simulink model "BungeeJumpingDragSoln"  (R2024a)
settings: Solver=VariableStepAuto  StartTime=0.0  StopTime=50  MaxStep=0.1  RelTol=1e-3
PreLoadFcn:
  | load Data\BungeeParamsDrag.mat
undefined symbols (not defined in the file): A, Cd, g, k, L, m, rho, x0
CloseFcn:
  | clear
settings Model: Creator=callie  LastModifiedBy=callie
settings DataIOCC: ReturnWorkspaceOutputsName=out2

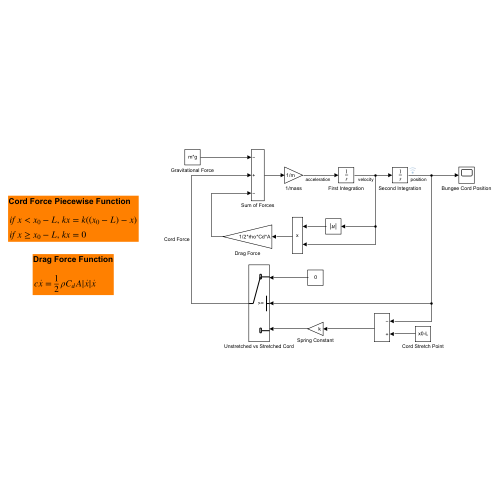
[thumbnail: Simulink's stored preview of the top-level diagram]
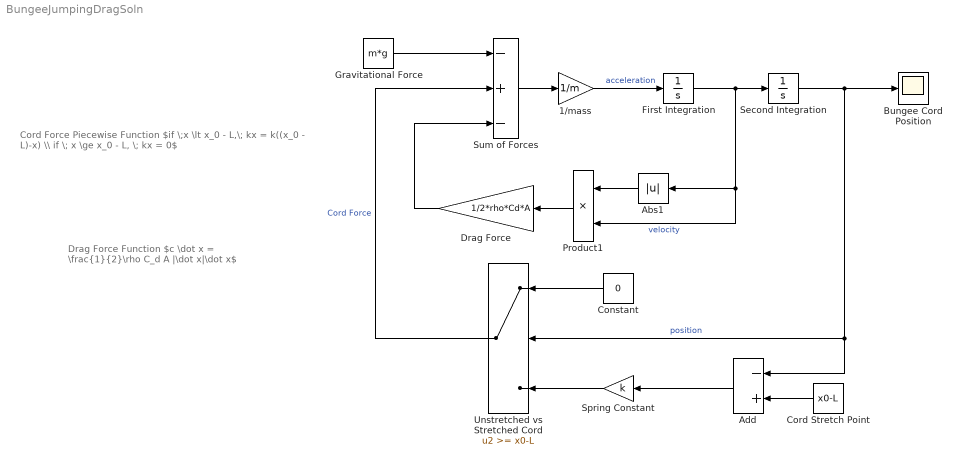
== system BungeeJumpingDragSoln ==
  note: Drag Force Function
      |
      | $c \dot x = \frac{1}{2}\rho C_d A |\dot x|\dot x$
  note: Cord Force Piecewise Function
      |
      | $if \;x \lt x_0 - L,\; kx = k((x_0 - L)-x) \\ if \; x \ge x_0 - L, \; kx = 0$
  1/mass : Gain  Gain=1/m  SaturateOnIntegerOverflow=on  OutDataTypeStr=Inherit: Same as input  ParamDataTypeStr=Inherit: Same as input
  Abs1 : Abs  SaturateOnIntegerOverflow=off
  Add : Sum  Inputs=-+
  Bungee Cord Position : Scope
  Constant : Constant  Value=0
  Cord Stretch Point : Constant  Value=x0-L
  Drag Force : Gain  Gain=1/2*rho*Cd*A
  First Integration : Integrator
  Gravitational Force : Constant  Value=m*g
  Product1 : Product  RndMeth=Zero
  Second Integration : Integrator  InitialCondition=x0
  Spring Constant : Gain  Gain=k  SaturateOnIntegerOverflow=on  OutDataTypeStr=Inherit: Same as input  ParamDataTypeStr=Inherit: Same as input
  Sum of Forces : Sum  Inputs=-+-  InputSameDT=on  SaturateOnIntegerOverflow=on  OutDataTypeStr=Inherit: Same as first input
  Unstretched vs Stretched Cord : Switch  Threshold=x0-L
  wires:
  Sum of Forces/1 -> 1/mass/1
  Second Integration/1 -> Unstretched vs Stretched Cord/2, Add/1, Bungee Cord Position/1  "position"
  Unstretched vs Stretched Cord/1 -> Sum of Forces/2  "Cord Force"
  Cord Stretch Point/1 -> Add/2
  Add/1 -> Spring Constant/1
  Spring Constant/1 -> Unstretched vs Stretched Cord/3
  Gravitational Force/1 -> Sum of Forces/1
  1/mass/1 -> First Integration/1  "acceleration"
  Constant/1 -> Unstretched vs Stretched Cord/1
  Abs1/1 -> Product1/1
  First Integration/1 -> Abs1/1, Product1/2, Second Integration/1  "velocity"
  Product1/1 -> Drag Force/1
  Drag Force/1 -> Sum of Forces/3
